simulink model "model_zaworGora"  (R2015a)
settings: Solver=ode4  StartTime=0.0  StopTime=T_sim  FixedStep=0.1  RelTol=1e-3
values from neighbouring files (symbols this model uses):
  h0 = poziom(1)    [chka_zawor_gora.m]
  p1 = polyfit(PWM_level, pred_napelniania, 2)    [chka_zawor_gora.m]    (also in skryptDoIdentyfikacji.m = [-49.142857142857010 99.114285714285490 -23.369999999999905]; wskaznikJakosci.m = [-49.142857142857010 99.114285714285490 -23.369999999999905])
  pC2 = polyfit(PWM_level_C2, C2, 2)    [chka_zawor_gora.m]
  PWM = 0.4    [chka_zawor_gora.m]    (also in skryptDoIdentyfikacji.m = 1; wskaznikJakosci.m = 1)
settings Model: Creator=konra  LastModifiedBy=konra
settings DataIOCC: LimitDataPoints=off

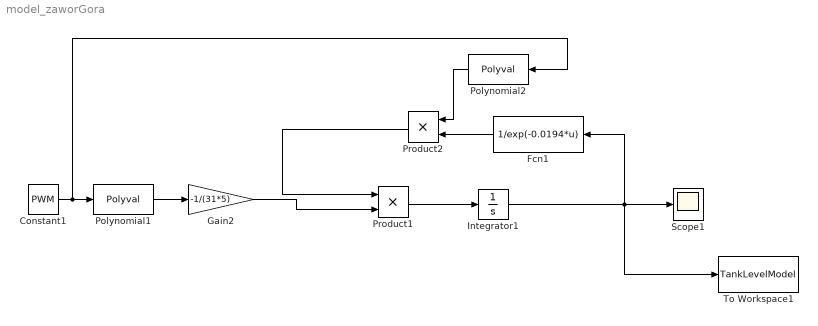
== system model_zaworGora ==
  Constant1 : Constant  Value=PWM
  Fcn1 : Fcn  Expr=1/exp(-0.0194*u)
  Gain2 : Gain  Gain=-1/(31*5)
  Integrator1 : Integrator  InitialCondition=h0
  Polynomial1 : Polyval  Coefs=p1
  Polynomial2 : Polyval  Coefs=pC2
  Product1 : Product
  Product2 : Product
  Scope1 : Scope
      settings: TimeRange=180
  To Workspace1 : ToWorkspace  VariableName=TankLevelModel  SaveFormat=Structure With Time  SampleTime=-1
  wires:
  Polynomial1/1 -> Gain2/1
  Gain2/1 -> Product1/2
  Product1/1 -> Integrator1/1
  Fcn1/1 -> Product2/2
  Product2/1 -> Product1/1
  Constant1/1 -> Polynomial2/1, Polynomial1/1
  Polynomial2/1 -> Product2/1
  Integrator1/1 -> Fcn1/1, Scope1/1, To Workspace1/1
